simulink model "Cell_Balancing_Using_Passive_Method_Static_Condition"  (R2024a)
settings: Solver=VariableStepAuto  StartTime=0.0  StopTime=1180  RelTol=1e-3
libraries: simulink x4
settings Model: Creator=gopin  LastModifiedBy=gopin

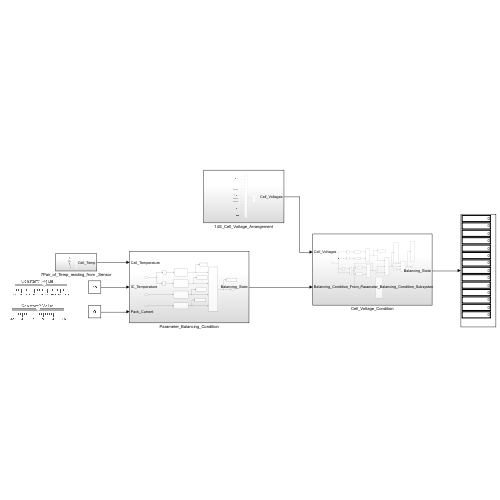
[thumbnail: Simulink's stored preview of the top-level diagram]
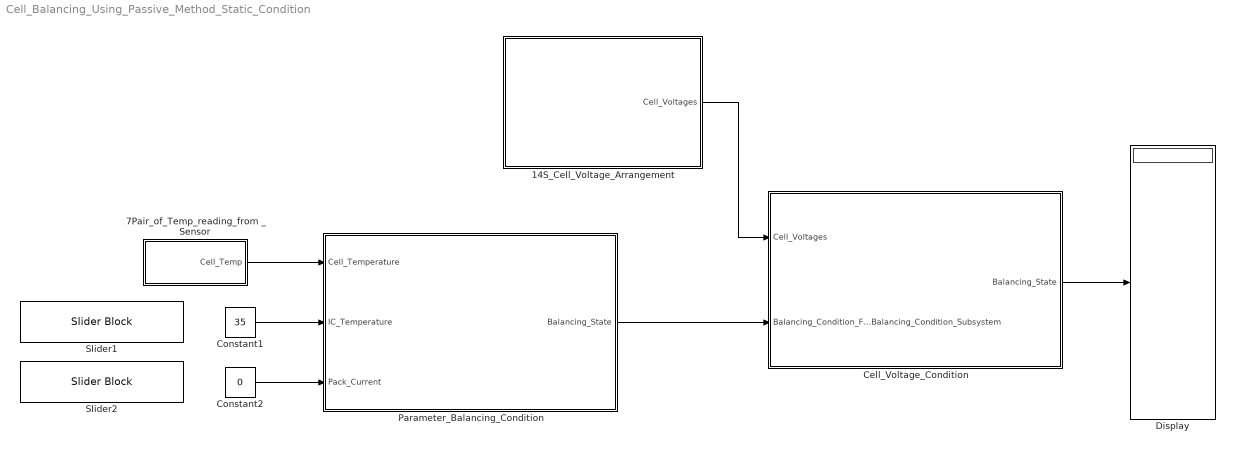
== system Cell_Balancing_Using_Passive_Method_Static_Condition ==
  14S_Cell_Voltage_Arrangement : Subsystem
  7Pair_of_Temp_reading_from _Sensor : Subsystem
  Cell_Voltage_Condition : Subsystem
  Constant1 : Constant  Value=35
  Constant2 : Constant  Value=0
  Display : Display
  Parameter_Balancing_Condition : Subsystem
  Slider1 : SliderBlock  ScaleMin=-10  ScaleMax=70
  Slider2 : SliderBlock  ScaleMin=-10  ScaleMax=10
  wires:
  Constant1/1 -> Parameter_Balancing_Condition/2(IC_Temperature)
  Parameter_Balancing_Condition/1(Balancing_State) -> Cell_Voltage_Condition/2(Balancing_Condition_From_Parameter_Balancing_Condition_Subsystem)
  Constant2/1 -> Parameter_Balancing_Condition/3(Pack_Current)
  Cell_Voltage_Condition/1(Balancing_State) -> Display/1
  14S_Cell_Voltage_Arrangement/1(Cell_Voltages) -> Cell_Voltage_Condition/1(Cell_Voltages)
  7Pair_of_Temp_reading_from _Sensor/1(Cell_Temp) -> Parameter_Balancing_Condition/1(Cell_Temperature)

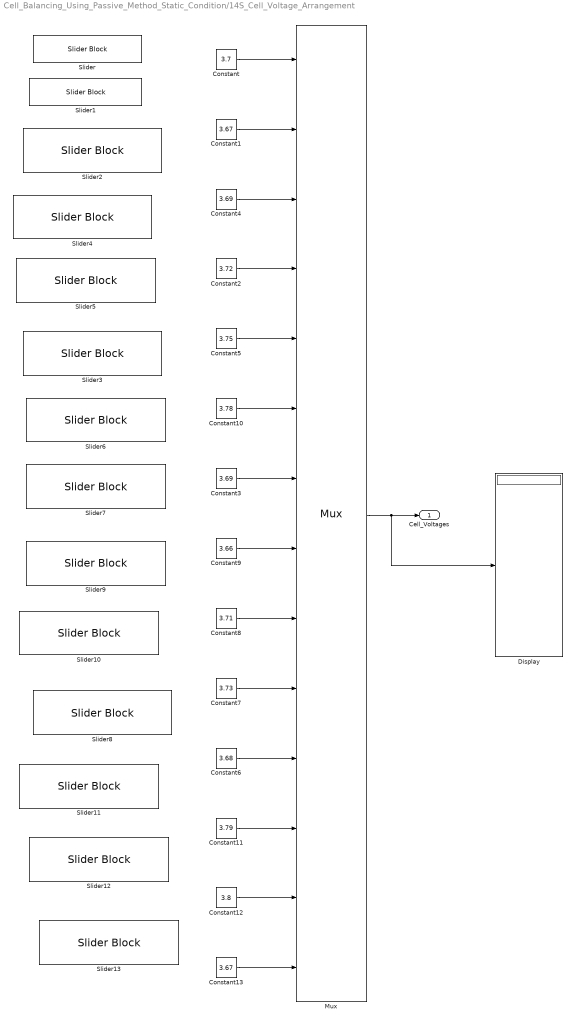
== system Cell_Balancing_Using_Passive_Method_Static_Condition/14S_Cell_Voltage_Arrangement ==
  Constant : Constant  Value=3.7
  Constant1 : Constant  Value=3.67
  Constant10 : Constant  Value=3.78
  Constant11 : Constant  Value=3.79
  Constant12 : Constant  Value=3.8
  Constant13 : Constant  Value=3.67
  Constant2 : Constant  Value=3.72
  Constant3 : Constant  Value=3.69
  Constant4 : Constant  Value=3.69
  Constant5 : Constant  Value=3.75
  Constant6 : Constant  Value=3.68
  Constant7 : Constant  Value=3.73
  Constant8 : Constant  Value=3.71
  Constant9 : Constant  Value=3.66
  Display : Display
  Mux : Mux  Inputs=14
  Slider{,1..13} (14 alike) : SliderBlock  ScaleMin=2.5  ScaleMax=4.25
  Cell_Voltages : Outport
  wires:
  Constant/1 -> Mux/1
  Constant1/1 -> Mux/2
  Constant4/1 -> Mux/3
  Constant2/1 -> Mux/4
  Constant5/1 -> Mux/5
  Constant10/1 -> Mux/6
  Constant3/1 -> Mux/7
  Constant9/1 -> Mux/8
  Constant8/1 -> Mux/9
  Constant7/1 -> Mux/10
  Constant6/1 -> Mux/11
  Constant11/1 -> Mux/12
  Constant12/1 -> Mux/13
  Constant13/1 -> Mux/14
  Mux/1 -> Display/1, Cell_Voltages/1

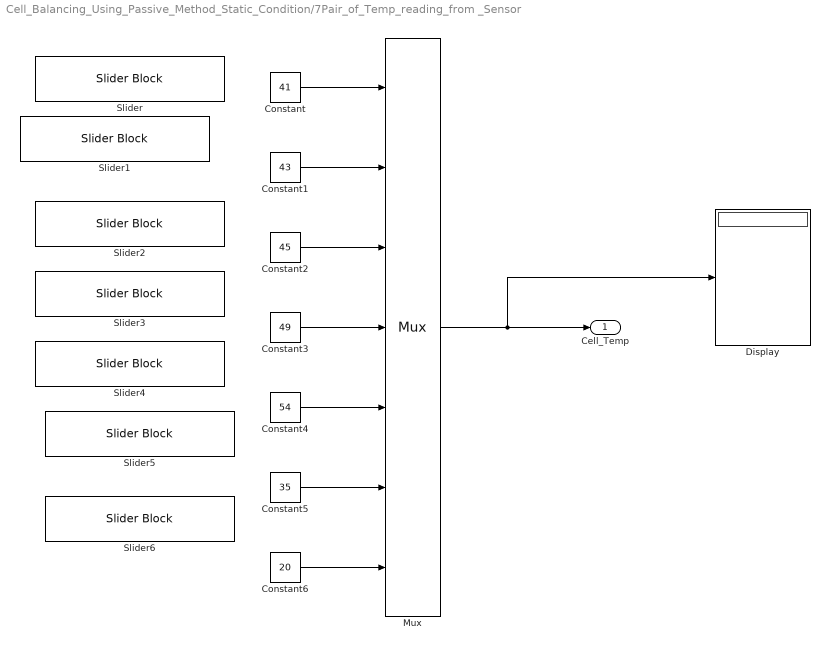
== system Cell_Balancing_Using_Passive_Method_Static_Condition/7Pair_of_Temp_reading_from _Sensor ==
  Constant : Constant  Value=41
  Constant1 : Constant  Value=43
  Constant2 : Constant  Value=45
  Constant3 : Constant  Value=49
  Constant4 : Constant  Value=54
  Constant5 : Constant  Value=35
  Constant6 : Constant  Value=20
  Display : Display
  Mux : Mux  Inputs=7
  Slider{,1..6} (7 alike) : SliderBlock  ScaleMin=-10  ScaleMax=70
  Cell_Temp : Outport
  wires:
  Mux/1 -> Display/1, Cell_Temp/1
  Constant/1 -> Mux/1
  Constant1/1 -> Mux/2
  Constant2/1 -> Mux/3
  Constant3/1 -> Mux/4
  Constant4/1 -> Mux/5
  Constant5/1 -> Mux/6
  Constant6/1 -> Mux/7

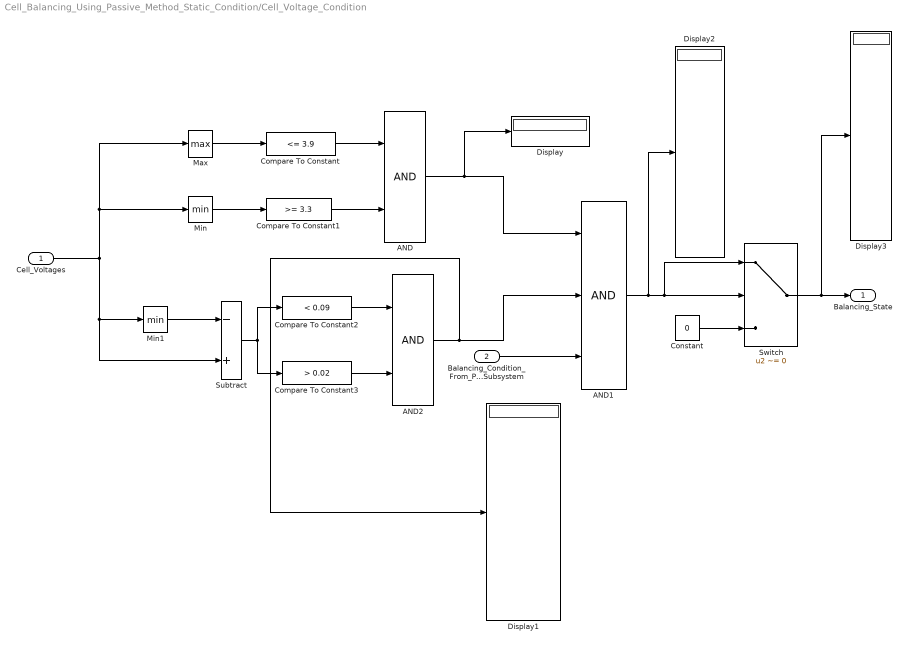
== system Cell_Balancing_Using_Passive_Method_Static_Condition/Cell_Voltage_Condition ==
  Cell_Voltages : Inport
  Balancing_Condition_From_Parameter_Balancing_Condition_Subsystem : Inport  Port=2
  AND : Logic  AllPortsSameDT=off  OutDataTypeStr=boolean
  AND1 : Logic  Inputs=3  AllPortsSameDT=off  OutDataTypeStr=boolean
  AND2 : Logic  AllPortsSameDT=off  OutDataTypeStr=boolean
  Compare To Constant : simulink/Logic and Bit Operations/Compare To Constant  relop=<=  const=3.9  OutDataTypeStr=boolean
  Compare To Constant1 : simulink/Logic and Bit Operations/Compare To Constant  relop=>=  const=3.3  OutDataTypeStr=boolean
  Compare To Constant2 : simulink/Logic and Bit Operations/Compare To Constant  relop=<  const=0.09  OutDataTypeStr=boolean
  Compare To Constant3 : simulink/Logic and Bit Operations/Compare To Constant  relop=>  const=0.02  OutDataTypeStr=boolean
  Constant : Constant  Value=0
  Display{,1..3} (4 alike) : Display
  Max : MinMax  Function=max
  Min : MinMax
  Min1 : MinMax
  Subtract : Sum  Inputs=-+
  Switch : Switch  Criteria=u2 ~= 0  SaturateOnIntegerOverflow=off  InputSameDT=off
  Balancing_State : Outport
  wires:
  Cell_Voltages/1 -> Max/1, Min/1, Subtract/2, Min1/1
  Max/1 -> Compare To Constant/1
  Min/1 -> Compare To Constant1/1
  Compare To Constant/1 -> AND/1
  Compare To Constant1/1 -> AND/2
  AND/1 -> Display/1, AND1/1
  AND2/1 -> Display1/1, AND1/2
  Min1/1 -> Subtract/1
  Subtract/1 -> Compare To Constant3/1, Compare To Constant2/1
  Compare To Constant2/1 -> AND2/1
  Compare To Constant3/1 -> AND2/2
  Switch/1 -> Display3/1, Balancing_State/1
  AND1/1 -> Display2/1, Switch/1, Switch/2
  Balancing_Condition_From_Parameter_Balancing_Condition_Subsystem/1 -> AND1/3
  Constant/1 -> Switch/3

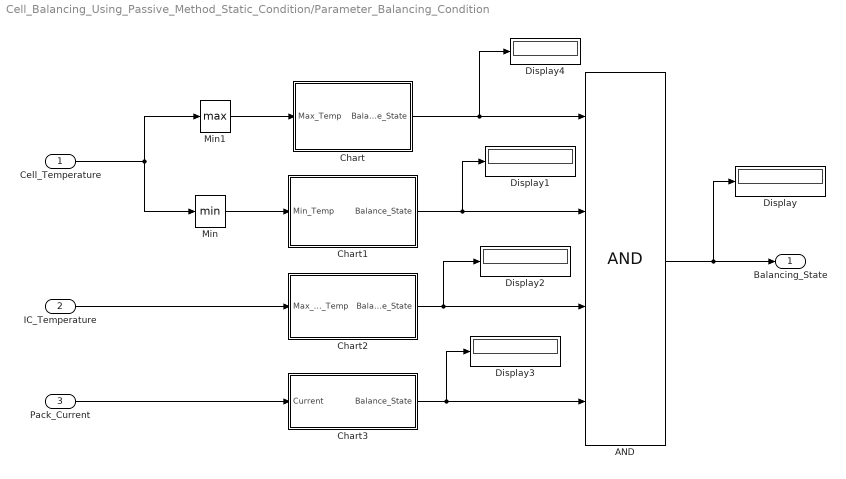
== system Cell_Balancing_Using_Passive_Method_Static_Condition/Parameter_Balancing_Condition ==
  Cell_Temperature : Inport
  IC_Temperature : Inport  Port=2
  Pack_Current : Inport  Port=3
  AND : Logic  Inputs=4  AllPortsSameDT=off  OutDataTypeStr=boolean
  Chart : Stateflow chart  TreatAsAtomicUnit=on
  Chart1 : Stateflow chart  TreatAsAtomicUnit=on
  Chart2 : Stateflow chart  TreatAsAtomicUnit=on
  Chart3 : Stateflow chart  TreatAsAtomicUnit=on
  Display{,1..4} (5 alike) : Display
  Min : MinMax
  Min1 : MinMax  Function=max
  Balancing_State : Outport
  wires:
  Cell_Temperature/1 -> Min1/1, Min/1
  AND/1 -> Display/1, Balancing_State/1
  Min1/1 -> Chart/1(Max_Temp)
  Min/1 -> Chart1/1(Min_Temp)
  Chart1/1(Balance_State) -> Display1/1, AND/2
  Chart/1(Balance_State) -> Display4/1, AND/1
  IC_Temperature/1 -> Chart2/1(Max_IC_Temp)
  Chart2/1(Balance_State) -> Display2/1, AND/3
  Pack_Current/1 -> Chart3/1(Current)
  Chart3/1(Balance_State) -> Display3/1, AND/4

== stateflow chart Cell_Balancing_Using_Passive_Method_Static_Condition/Parameter_Balancing_Condition/Chart1 ==
  state Balance_Condition_1
    en:
    Balance_State=1;
  state Balance_Condition_2
    en:
    Balance_State=0;
  (default) -> Balance_Condition_1
  Balance_Condition_1 -> Balance_Condition_2 : [Min_Temp<10]
  Balance_Condition_2 -> Balance_Condition_1 : [Min_Temp>=15]
  data: Min_Temp input; Balance_State output

== stateflow chart Cell_Balancing_Using_Passive_Method_Static_Condition/Parameter_Balancing_Condition/Chart2 ==
  state Balance_Condition_1
    en:
    Balance_State=1;
  state Balance_Condition_2
    en:
    Balance_State=0;
  (default) -> Balance_Condition_1
  Balance_Condition_1 -> Balance_Condition_2 : [Max_IC_Temp>60]
  Balance_Condition_2 -> Balance_Condition_1 : [Max_IC_Temp<=50]
  data: Max_IC_Temp input; Balance_State output

== stateflow chart Cell_Balancing_Using_Passive_Method_Static_Condition/Parameter_Balancing_Condition/Chart ==
  state Balance_Condition_1
    en:
    Balance_State=1;
  state Balance_Condition_2
    en:
    Balance_State=0;
  (default) -> Balance_Condition_1
  Balance_Condition_1 -> Balance_Condition_2 : [Max_Temp>50]
  Balance_Condition_2 -> Balance_Condition_1 : [Max_Temp<=40]
  data: Balance_State output; Max_Temp input

== stateflow chart Cell_Balancing_Using_Passive_Method_Static_Condition/Parameter_Balancing_Condition/Chart3 ==
  state Balance_Condition_1
    en:
    Balance_State=1;
  state Balance_Condition_2
    en:
    Balance_State=0;
  (default) -> Balance_Condition_1
  Balance_Condition_1 -> Balance_Condition_2 : [Current>1 || Current<-1]
  Balance_Condition_2 -> Balance_Condition_1 : [Current<1 && Current>-1]
  data: Balance_State output; Current input
